simulink model "M17_Q4"  (R2017a)
settings: Solver=ode4  StartTime=0.0  StopTime=2500  FixedStep=STEP_SIZE  RelTol=1e-3  EnableMultiTasking=on
undefined symbols (not defined in the file): b, Bv, c, f, g, K, M, offset, p, rhoa0, stoc, Ta0, tau1, tc, us400, V, V1, V2, xs400
libraries: simulink x2
settings Model: Creator=Mikkel  LastModifiedBy=Roberto
settings DataIOCC: LimitDataPoints=on  SaveFormat=Array  SignalLoggingSaveFormat=ModelDataLogs
settings OptimizationCC: ExpressionDepthLimit=2147483647  LifeSpan=inf
settings DebuggingCC: UnderspecifiedInitializationDetection=Classic  MergeDetectMultiDrivingBlocksExec=none  FcnCallInpInsideContextMsg=warning  StateNameClashWarn=warning  SFUnexpectedBacktrackingDiag=warning  SFNoUnconditionalDefaultTransitionDiag=warning  SFExecutionAtInitializationDiag=none
settings HardwareCC: ProdBitPerPointer=32  ProdBitPerSizeT=32  ProdBitPerPtrDiffT=32  ProdLargestAtomicFloat=None  ProdIntDivRoundTo=Undefined  ProdEndianess=Unspecified  ProdWordSize=32  ProdHWDeviceType=32-bit Generic
settings ModelReferenceCC: PropagateSignalLabelsOutOfModel=off
settings GRTTargetCC: TargetLangStandard=C89/C90 (ANSI)  CombineOutputUpdateFcns=off  GRTInterface=on
settings ConfigComp: CovMetricSettings=dw  CovHtmlReporting=on  CovSaveCumulativeToWorkspaceVar=on  CovSaveSingleToWorkspaceVar=on  CovExternalEMLEnable=off

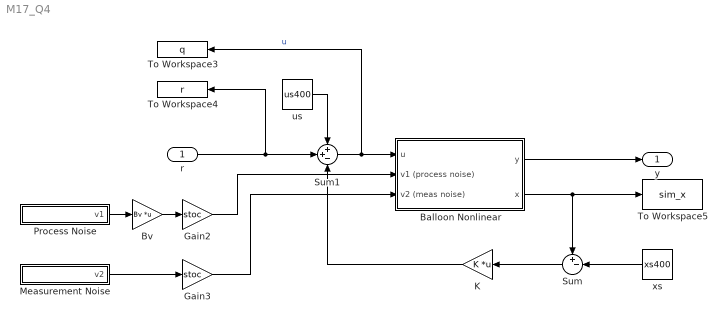
== system M17_Q4 ==
  r : Inport
  Balloon Nonlinear : Subsystem
  Bv : Gain  Gain=Bv  Multiplication=Matrix(K*u)
  Gain2 : Gain  Gain=stoc
  Gain3 : Gain  Gain=stoc
  K : Gain  Gain=K  Multiplication=Matrix(K*u)
  Measurement Noise : Subsystem
  Process Noise : Subsystem
  Sum : Sum  Inputs=+-|
  Sum1 : Sum  Inputs=++-
  To Workspace3 : ToWorkspace  VariableName=q  SaveFormat=Structure With Time  SampleTime=-1
  To Workspace4 : ToWorkspace  VariableName=r  SaveFormat=Structure With Time  SampleTime=-1
  To Workspace5 : ToWorkspace  VariableName=sim_x  SaveFormat=Structure With Time  SampleTime=-1
  us : Constant  Value=us400
  xs : Constant  Value=xs400
  y : Outport
  wires:
  r/1 -> Sum1/2, To Workspace4/1
  Balloon Nonlinear/2(x) -> Sum/1, To Workspace5/1
  xs/1 -> Sum/2
  Sum/1 -> K/1
  Sum1/1 -> Balloon Nonlinear/1(u), To Workspace3/1  "u"
  Balloon Nonlinear/1(y) -> y/1
  Gain2/1 -> Balloon Nonlinear/2(v1 (process noise))
  Gain3/1 -> Balloon Nonlinear/3(v2 (meas noise))
  Bv/1 -> Gain2/1
  Process Noise/1(v1) -> Bv/1
  Measurement Noise/1(v2) -> Gain3/1
  K/1 -> Sum1/3
  us/1 -> Sum1/1

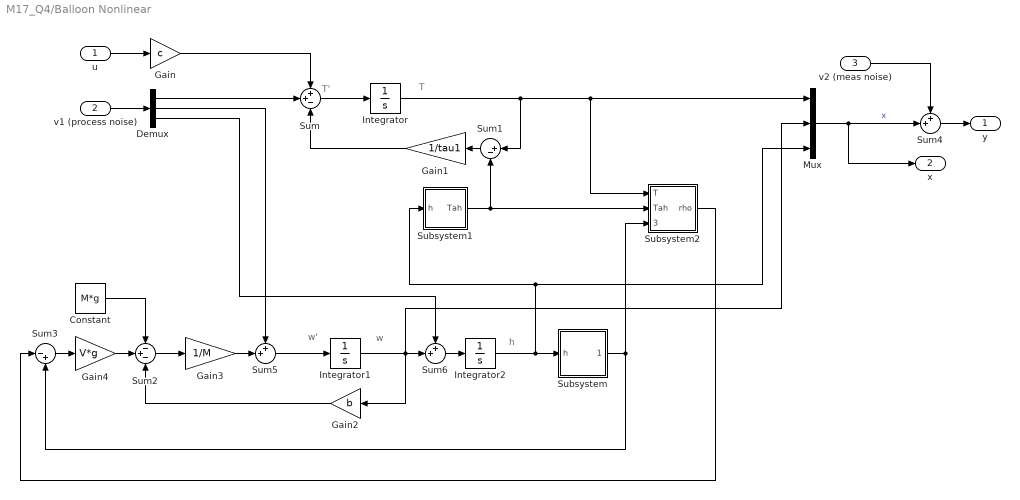
== system M17_Q4/Balloon Nonlinear ==
  note: T
  note: T'
  note: w
  note: w'
  note: h
  u : Inport
  v1 (process noise) : Inport  Port=2
  v2 (meas noise) : Inport  Port=3
  Constant : Constant  Value=M*g
  Demux : Demux  Outputs=3
  Gain : Gain  Gain=c
  Gain1 : Gain  Gain=1/tau1
  Gain2 : Gain  Gain=b
  Gain3 : Gain  Gain=1/M
  Gain4 : Gain  Gain=V*g
  Integrator : Integrator  Priority=1  InitialCondition=xs400(1)
  Integrator1 : Integrator  Priority=2  InitialCondition=xs400(2)
  Integrator2 : Integrator  Priority=3  InitialCondition=xs400(3)
  Mux : Mux  Inputs=3
  Subsystem : Subsystem
  Subsystem1 : Subsystem
  Subsystem2 : Subsystem
  Sum : Sum  Inputs=++-
  Sum1 : Sum  Inputs=|+-
  Sum2 : Sum  Inputs=-+-
  Sum3 : Sum  Inputs=|-+
  Sum4 : Sum  Inputs=++|
  Sum5 : Sum  Inputs=++|
  Sum6 : Sum  Inputs=++|
  y : Outport
  x : Outport  Port=2
  wires:
  Integrator2/1 -> Subsystem1/1(h), Mux/3, Subsystem/1(h)
  Subsystem/1(rhoah) -> Subsystem2/3(rhoah), Sum3/2
  Gain4/1 -> Sum2/2
  Integrator/1 -> Sum1/1, Mux/1, Subsystem2/1(T)
  Sum2/1 -> Gain3/1
  Sum1/1 -> Gain1/1
  Subsystem1/1(Tah) -> Sum1/2, Subsystem2/2(Tah)
  Integrator1/1 -> Sum6/2, Gain2/1, Mux/2
  Gain2/1 -> Sum2/3
  Subsystem2/1(rho) -> Sum3/1
  Sum/1 -> Integrator/1
  Sum3/1 -> Gain4/1
  Constant/1 -> Sum2/1
  Mux/1 -> Sum4/2, x/1  "x"
  u/1 -> Gain/1
  Sum4/1 -> y/1
  v2 (meas noise)/1 -> Sum4/1
  v1 (process noise)/1 -> Demux/1
  Gain1/1 -> Sum/3
  Gain/1 -> Sum/1
  Demux/1 -> Sum/2
  Gain3/1 -> Sum5/2
  Sum5/1 -> Integrator1/1
  Demux/2 -> Sum5/1
  Sum6/1 -> Integrator2/1
  Demux/3 -> Sum6/1

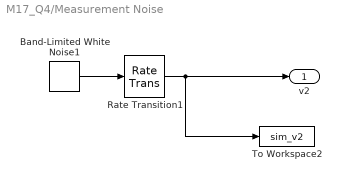
== system M17_Q4/Measurement Noise ==
  Band-Limited White Noise1 : simulink/Sources/Band-Limited White Noise  Cov=diag(V2)  Ts=tc  seed=[4702 44280 1342]
  Rate Transition1 : RateTransition  OutPortSampleTimeOpt=Inherit
  To Workspace2 : ToWorkspace  VariableName=sim_v2  SaveFormat=Structure With Time  SampleTime=-1
  v2 : Outport
  wires:
  Rate Transition1/1 -> v2/1, To Workspace2/1
  Band-Limited White Noise1/1 -> Rate Transition1/1

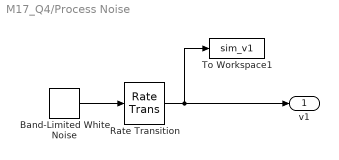
== system M17_Q4/Process Noise ==
  Band-Limited White Noise : simulink/Sources/Band-Limited White Noise  Cov=diag(V1)  Ts=tc  seed=[4892 2694 10842]
  Rate Transition : RateTransition  OutPortSampleTimeOpt=Inherit
  To Workspace1 : ToWorkspace  VariableName=sim_v1  SaveFormat=Structure With Time  SampleTime=-1
  v1 : Outport
  wires:
  Band-Limited White Noise/1 -> Rate Transition/1
  Rate Transition/1 -> v1/1, To Workspace1/1

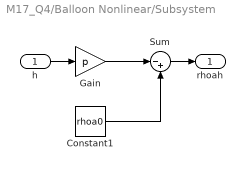
== system M17_Q4/Balloon Nonlinear/Subsystem ==
  h : Inport
  Constant1 : Constant  Value=rhoa0
  Gain : Gain  Gain=p
  Sum : Sum  Inputs=|-+
  rhoah : Outport
  wires:
  Constant1/1 -> Sum/2
  Gain/1 -> Sum/1
  h/1 -> Gain/1
  Sum/1 -> rhoah/1

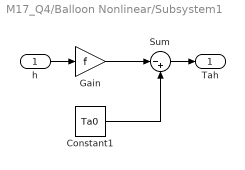
== system M17_Q4/Balloon Nonlinear/Subsystem1 ==
  h : Inport
  Constant1 : Constant  Value=Ta0
  Gain : Gain  Gain=f
  Sum : Sum  Inputs=|-+
  Tah : Outport
  wires:
  Constant1/1 -> Sum/2
  Gain/1 -> Sum/1
  h/1 -> Gain/1
  Sum/1 -> Tah/1

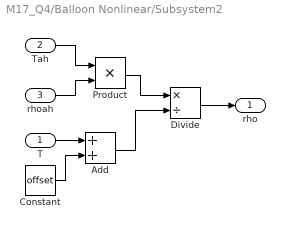
== system M17_Q4/Balloon Nonlinear/Subsystem2 ==
  T : Inport
  Tah : Inport  Port=2
  rhoah : Inport  Port=3
  Add : Sum
  Constant : Constant  Value=offset
  Divide : Product  Inputs=*/
  Product : Product  RndMeth=Zero
  rho : Outport
  wires:
  rhoah/1 -> Product/2
  Tah/1 -> Product/1
  Product/1 -> Divide/1
  Divide/1 -> rho/1
  Add/1 -> Divide/2
  T/1 -> Add/1
  Constant/1 -> Add/2
